simulink model "modelo_cinematico_movil"  (R2016b)
settings: Solver=VariableStepAuto  StartTime=0.0  StopTime=t_sim  RelTol=1e-3
values from neighbouring files (symbols this model uses):
  freq = input(selection)    [pruebas_MCD.m]    (also in pruebas_modelo.m = 0.25)
  omega = in(2)    [MCD_movil.m]    (also in MCI_movil.m = jac_inv(2,:)*gen; control_linea.m = -Kd*d+Kh*err_ang; control_persecucion.m = v_ref/R; control_tray.m = Kh*(phi_ref-phi))
  omega_sat = [-0.2618 0.2618]    [prueba_persecucionPURA.m]    (also in pruebas_MCD.m; pruebas_MCI.m; pruebas_control.m; pruebas_control_P2.m)
  pos_init = [0;0;0]    [prueba_persecucionPURA.m]    (also in pruebas_MCD.m; pruebas_MCI.m; pruebas_control.m; pruebas_control_P2.m)
  tetha_d = in(1)    [MCD_movil.m]    (also in MCI_movil.m = jac_inv(1,:)*gen; pruebas_MCD.m = tetha_d_sat(1); pruebas_modelo.m = 5)
  tetha_d_sat = [-0.75 0.75]    [prueba_persecucionPURA.m]    (also in pruebas_MCD.m; pruebas_MCI.m; pruebas_control.m; pruebas_control_P2.m)
settings Model: Creator=marrcogrova  LastModifiedBy=Javi Owo

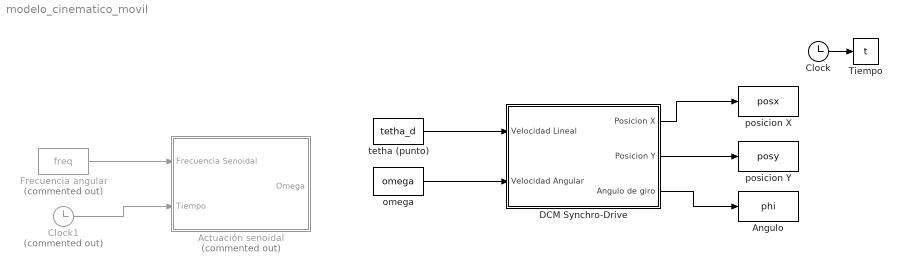
== system modelo_cinematico_movil ==
  Actuación senoidal : Subsystem  Commented=on
  Angulo : ToWorkspace  VariableName=phi  SampleTime=-1
  Clock : Clock
  Clock1 : Clock  Commented=on
  DCM Synchro-Drive : Subsystem
  Frecuencia angular : Constant  Commented=on  Value=freq
  Tiempo : ToWorkspace  VariableName=t  SampleTime=-1
  omega : Constant  Value=omega
  posicion X : ToWorkspace  VariableName=posx  SampleTime=-1
  posicion Y : ToWorkspace  VariableName=posy  SampleTime=-1
  tetha (punto) : Constant  Value=tetha_d
  wires:
  DCM Synchro-Drive/1(Posicion X) -> posicion X/1
  DCM Synchro-Drive/2(Posicion Y) -> posicion Y/1
  DCM Synchro-Drive/3(Angulo de giro) -> Angulo/1
  Clock/1 -> Tiempo/1
  tetha (punto)/1 -> DCM Synchro-Drive/1(Velocidad Lineal)
  Clock1/1 -> Actuación senoidal/2(Tiempo)
  Frecuencia angular/1 -> Actuación senoidal/1(Frecuencia Senoidal)
  omega/1 -> DCM Synchro-Drive/2(Velocidad Angular)

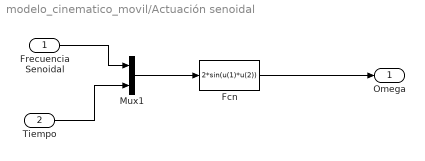
== system modelo_cinematico_movil/Actuación senoidal ==
  Frecuencia Senoidal : Inport
  Tiempo : Inport  Port=2
  Fcn : Fcn  Expr=2*sin(u(1)*u(2))
  Mux1 : Mux  Inputs=2
  Omega : Outport
  wires:
  Fcn/1 -> Omega/1
  Frecuencia Senoidal/1 -> Mux1/1
  Mux1/1 -> Fcn/1
  Tiempo/1 -> Mux1/2

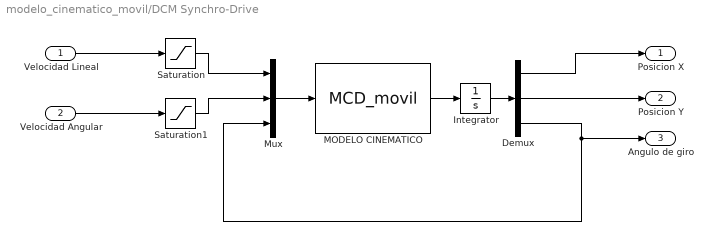
== system modelo_cinematico_movil/DCM Synchro-Drive ==
  Velocidad Lineal : Inport
  Velocidad Angular : Inport  Port=2
  Demux : Demux  Outputs=3
  Integrator : Integrator  InitialCondition=pos_init
  MODELO CINEMATICO : MATLABFcn  MATLABFcn=MCD_movil  OutputDimensions=3
  Mux : Mux  Inputs=3
  Saturation : Saturate  UpperLimit=tetha_d_sat(2)  LowerLimit=tetha_d_sat(1)
  Saturation1 : Saturate  UpperLimit=omega_sat(2)  LowerLimit=omega_sat(1)
  Posicion X : Outport
  Posicion Y : Outport  Port=2
  Angulo de giro : Outport  Port=3
  wires:
  Integrator/1 -> Demux/1
  Demux/3 -> Angulo de giro/1, Mux/3
  Demux/1 -> Posicion X/1
  Demux/2 -> Posicion Y/1
  Mux/1 -> MODELO CINEMATICO/1
  MODELO CINEMATICO/1 -> Integrator/1
  Velocidad Lineal/1 -> Saturation/1
  Saturation/1 -> Mux/1
  Saturation1/1 -> Mux/2
  Velocidad Angular/1 -> Saturation1/1
